simulink model "hdl_model_fixed"  (R2024a)
settings: Solver=VariableStepAuto  StartTime=0.0  StopTime=2  RelTol=1e-3
values from neighbouring files (symbols this model uses):
  BUFFER_LEN = 2048    [workspace.mat]
  SAMPLING_FREQ = 12800    [workspace.mat]
  signal_1 = [0 0.0001 0.0002 0.0003 0.0004 0.0005 0.0006 0.0007 0.0008 0.0009 0.001 0.0011 ... (4096 elements, 2048x2)]    [workspace.mat]
libraries: hdlsllib x2, dspsrcs4 x1, dsphdlxfrm2 x1, simulink_extras x1, dspsigops x1
settings Model: SimulationMode=accelerator  Creator=Jan Rosa  LastModifiedBy=Jan Rosa
settings DebuggingCC: SignalRangeChecking=warning

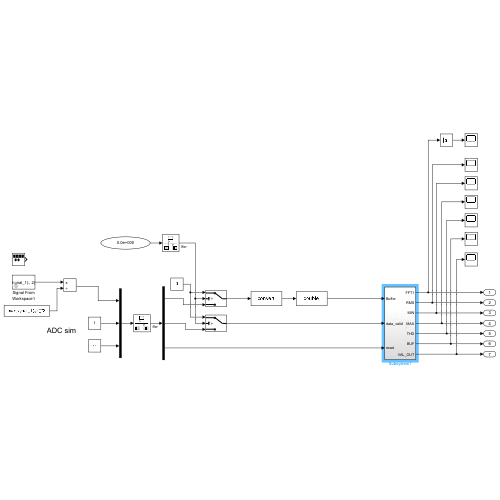
[thumbnail: Simulink's stored preview of the top-level diagram]
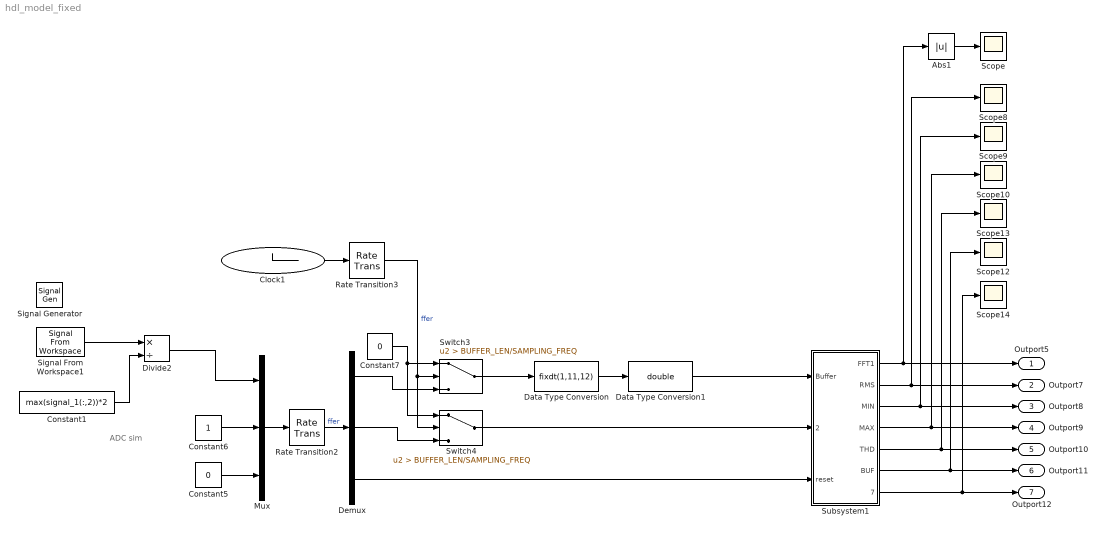
== system hdl_model_fixed ==
  note: ADC sim
  Abs1 : Abs  SaturateOnIntegerOverflow=off
  Clock1 : Clock
  Constant1 : Constant  Value=max(signal_1(:,2))*2
  Constant5 : Constant  Value=0
  Constant6 : Constant
  Constant7 : Constant  Value=0  SampleTime=1/SAMPLING_FREQ
  Data Type Conversion : DataTypeConversion  OutDataTypeStr=fixdt(1,11,12)  SaturateOnIntegerOverflow=off  RndMeth=Floor  LockScale=on
  Data Type Conversion1 : DataTypeConversion  OutDataTypeStr=double  SaturateOnIntegerOverflow=off  RndMeth=Floor
  Demux : Demux  Outputs=3
  Divide2 : Product  Inputs=*/
  Mux : Mux  Inputs=3
  Rate Transition2 : RateTransition  Integrity=off  Deterministic=off  OutPortSampleTime=1/SAMPLING_FREQ
  Rate Transition3 : RateTransition  Integrity=off  Deterministic=off  OutPortSampleTime=1/SAMPLING_FREQ
  Scope{,8..10,12..14} (7 alike) : Scope
  Signal Generator : SignalGenerator  WaveForm=square  Amplitude=0.49999  Frequency=50
  Signal From Workspace1 : dspsrcs4/Signal From Workspace  X=signal_1(:, 2)  Ts=signal_1(2, 1)  nsamps=1  OutputAfterFinalValue=Cyclic repetition  ignoreOrWarnInputAndFrameLengths=off  OutputFrames=off
  Subsystem1 : Subsystem
  Switch3 : Switch  Criteria=u2 > Threshold  Threshold=BUFFER_LEN/SAMPLING_FREQ  SaturateOnIntegerOverflow=off  InputSameDT=off
  Switch4 : Switch  Criteria=u2 > Threshold  Threshold=BUFFER_LEN/SAMPLING_FREQ  SaturateOnIntegerOverflow=off  InputSameDT=off
  Outport5 : Outport
  Outport7 : Outport  Port=2
  Outport8 : Outport  Port=3
  Outport9 : Outport  Port=4
  Outport10 : Outport  Port=5
  Outport11 : Outport  Port=6
  Outport12 : Outport  Port=7
  wires:
  Divide2/1 -> Mux/1
  Subsystem1/1(FFT1) -> Outport5/1, Abs1/1
  Switch4/1 -> Subsystem1/2(data_valid)
  Constant7/1 -> Switch4/1, Switch3/1
  Subsystem1/6(BUF) -> Outport11/1, Scope12/1
  Rate Transition3/1 -> Switch4/2, Switch3/2  "ffer"
  Subsystem1/7(VAL_OUT) -> Scope14/1, Outport12/1
  Subsystem1/4(MAX) -> Scope10/1, Outport9/1
  Demux/2 -> Switch4/3
  Clock1/1 -> Rate Transition3/1
  Demux/3 -> Subsystem1/3(reset)
  Subsystem1/5(THD) -> Scope13/1, Outport10/1
  Switch3/1 -> Data Type Conversion/1
  Demux/1 -> Switch3/3
  Mux/1 -> Rate Transition2/1
  Subsystem1/3(MIN) -> Scope9/1, Outport8/1
  Abs1/1 -> Scope/1
  Rate Transition2/1 -> Demux/1  "ffer"
  Constant5/1 -> Mux/3
  Signal From Workspace1/1 -> Divide2/1
  Constant6/1 -> Mux/2
  Constant1/1 -> Divide2/2
  Subsystem1/2(RMS) -> Outport7/1, Scope8/1
  Data Type Conversion/1 -> Data Type Conversion1/1
  Data Type Conversion1/1 -> Subsystem1/1(Buffer)

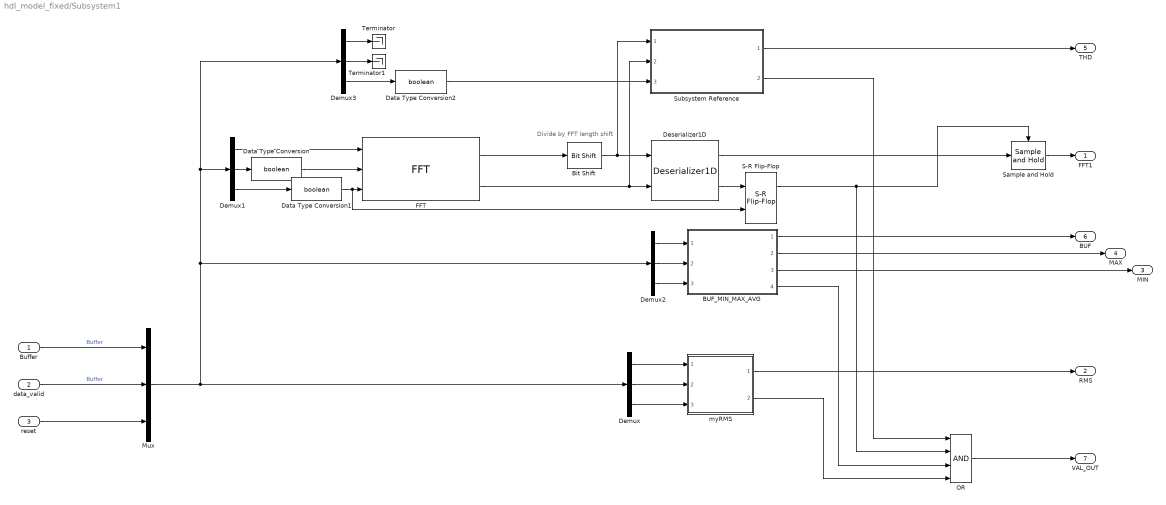
== system hdl_model_fixed/Subsystem1 ==
  note: Divide by FFT length shift
  Buffer : Inport
  data_valid : Inport  Port=2
  reset : Inport  Port=3
  BUF_MIN_MAX_AVG : Subsystem  ReferencedSubsystem=BUF_MIN_MAX_AVG_fixed
  Bit Shift : hdlsllib/Logic and Bit Operations/Bit Shift  mode=Shift Right Arithmetic  N=log2(BUFFER_LEN)
  Data Type Conversion : DataTypeConversion  OutDataTypeStr=boolean  SaturateOnIntegerOverflow=off  RndMeth=Floor
  Data Type Conversion1 : DataTypeConversion  OutDataTypeStr=boolean  SaturateOnIntegerOverflow=off  RndMeth=Floor
  Data Type Conversion2 : DataTypeConversion  OutDataTypeStr=boolean  SaturateOnIntegerOverflow=off  RndMeth=Floor
  Demux{,1..3} (4 alike) : Demux  Outputs=3
  Deserializer1D : hdlsllib/HDL Operations/Deserializer1D  Ratio=BUFFER_LEN  IdleCycles=0  InitialCondition=0  startIn=off  validIn=on  validOut=on  inputDataDimensions=-1  inputSampleTime=-1  inputSignalType=auto
  FFT : dsphdlxfrm2/FFT  Architecture=Streaming Radix 2^2  FFTLengthSource=Property  FFTLength=BUFFER_LEN  FFTLengthMax=1024  ComplexMultiplication=Use 4 multipliers and 2 adders  BitReversedOutput=off  BitReversedInput=off  Normalize=off  SimulateUsing=Code generation  RoundingMethod=Floor  ResetInputPort=on  StartOutputPort=off  EndOutputPort=off
  Mux : Mux  Inputs=3
  OR : Logic  Inputs=4  IconShape=distinctive  AllPortsSameDT=off  OutDataTypeStr=boolean
  S-R Flip-Flop : simulink_extras/Flip Flops/S-R Flip-Flop  initial_condition=0
  Sample and Hold : dspsigops/Sample and Hold  trig=Rising edge  initCond=0  latchinput=off
  Subsystem Reference : Subsystem  ReferencedSubsystem=myTHD_fixed
  Terminator : Terminator
  Terminator1 : Terminator
  myRMS : Subsystem  ReferencedSubsystem=myRMS_fixed
  FFT1 : Outport
  RMS : Outport  Port=2
  MIN : Outport  Port=3
  MAX : Outport  Port=4
  THD : Outport  Port=5
  BUF : Outport  Port=6
  VAL_OUT : Outport  Port=7
  wires:
  OR/1 -> VAL_OUT/1
  FFT/2 -> Subsystem Reference/2, Deserializer1D/2
  BUF_MIN_MAX_AVG/2 -> MAX/1
  BUF_MIN_MAX_AVG/3 -> MIN/1
  BUF_MIN_MAX_AVG/4 -> OR/3
  myRMS/1 -> RMS/1
  myRMS/2 -> OR/4
  Buffer/1 -> Mux/1  "Buffer"
  Demux/2 -> myRMS/2
  Demux/1 -> myRMS/1
  reset/1 -> Mux/3
  data_valid/1 -> Mux/2  "Buffer"
  Demux/3 -> myRMS/3
  Mux/1 -> Demux/1, Demux3/1, Demux1/1, Demux2/1
  Demux1/1 -> FFT/1
  Demux1/2 -> Data Type Conversion/1
  Demux1/3 -> Data Type Conversion1/1
  Demux2/1 -> BUF_MIN_MAX_AVG/1
  Demux2/2 -> BUF_MIN_MAX_AVG/2
  Demux2/3 -> BUF_MIN_MAX_AVG/3
  Demux3/3 -> Data Type Conversion2/1
  Demux3/1 -> Terminator/1
  Subsystem Reference/1 -> THD/1
  Subsystem Reference/2 -> OR/1
  Data Type Conversion1/1 -> S-R Flip-Flop/2, FFT/3
  Data Type Conversion/1 -> FFT/2
  Bit Shift/1 -> Deserializer1D/1, Subsystem Reference/1
  FFT/1 -> Bit Shift/1
  Deserializer1D/1 -> Sample and Hold/1
  Sample and Hold/1 -> FFT1/1
  Deserializer1D/2 -> S-R Flip-Flop/1
  S-R Flip-Flop/1 -> OR/2, Sample and Hold/Trigger
  Data Type Conversion2/1 -> Subsystem Reference/3
  Demux3/2 -> Terminator1/1
  BUF_MIN_MAX_AVG/1 -> BUF/1
